simulink model "exp1_1"  (R2018b)
settings: Solver=VariableStepAuto  StartTime=0.0  StopTime=100.0  RelTol=1e-3
settings Model: Creator=73  LastModifiedBy=73

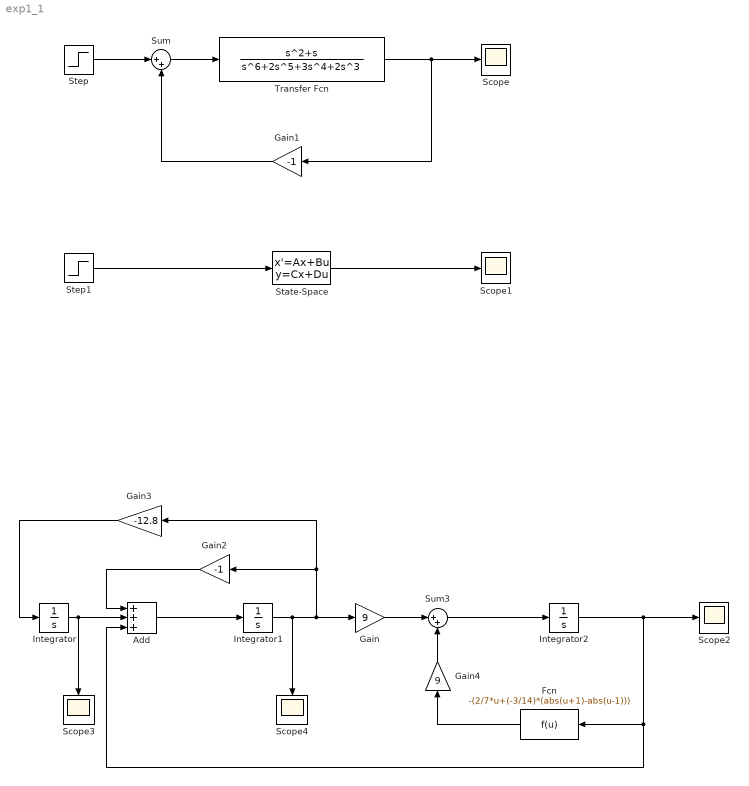
== system exp1_1 ==
  Add : Sum  Inputs=+++
  Fcn : Fcn  Expr=-(2/7*u+(-3/14)*(abs(u+1)-abs(u-1)))
  Gain : Gain  Gain=9
  Gain1 : Gain  Gain=-1
  Gain2 : Gain  Gain=-1
  Gain3 : Gain  Gain=-12.8
  Gain4 : Gain  Gain=9
  Integrator : Integrator  InitialCondition=0.7
  Integrator1 : Integrator  InitialCondition=0.3
  Integrator2 : Integrator  InitialCondition=-0.2
  Scope{,1..4} (5 alike) : Scope
  State-Space : StateSpace  A=[-2 -3 -2 -1 -1 0;1 0 0 0 0 0;0 1 0 0 0 0;0 0 1 0 0 0;0 0 0 1 0 0;0 0 0 0 1 0]  B=[1;0;0;0;0;0]  C=[0 0 0 1 1 0]  D=[0]  InitialCondition=0
  Step : Step  SampleTime=0
  Step1 : Step  SampleTime=0
  Sum : Sum  Inputs=|++
  Sum3 : Sum  Inputs=|++
  Transfer Fcn : TransferFcn  Numerator=[1 1 0]  Denominator=[1 2 3 2 0 0 0]
  wires:
  Step/1 -> Sum/1
  Gain1/1 -> Sum/2
  Sum/1 -> Transfer Fcn/1
  Transfer Fcn/1 -> Gain1/1, Scope/1
  Step1/1 -> State-Space/1
  State-Space/1 -> Scope1/1
  Sum3/1 -> Integrator2/1
  Integrator1/1 -> Gain3/1, Gain2/1, Gain/1, Scope4/1
  Gain/1 -> Sum3/1
  Fcn/1 -> Gain4/1
  Add/1 -> Integrator1/1
  Gain2/1 -> Add/1
  Integrator/1 -> Add/2, Scope3/1
  Gain3/1 -> Integrator/1
  Integrator2/1 -> Add/3, Fcn/1, Scope2/1
  Gain4/1 -> Sum3/2
